simulink model "controlScheme_UDP_4Beads"  (R2019b)
settings: Solver=FixedStepAuto  StartTime=0.0  StopTime=Inf  FixedStep=1/300  RelTol=1e-3  EnableMultiTasking=on
InitFcn:
  | tb = twinbeam('147.32.86.177', 30000);
  | 
  | tb.tracker_init(4);
  | pause(2)
  | 
  | tb.coords_subs(30006);
  | pause(1)
StopFcn:
  | delete(tb);
  | 
  | gen_udp = udp('147.32.86.177', 30001);
  | fopen(gen_udp);
  | fwrite(gen_udp, uint8('d'));
  | fclose(gen_udp);
  | delete(gen_udp);
model workspace (MAT data in the model file):
  NumberOfBeads = Simulink.Parameter
  NumberOfBeads.Value = 1
  NumberOfBeads.DataType = 'auto'
  NumberOfBeads.Dimensions = [1 1]
undefined symbols (not defined in the file): DiscIntNeverNeededParam, Joystick, Standard_Devices, UDP_Protocol
libraries: sldrtlib x3
settings Model: SimulationMode=accelerator  EnablePacing=on  ParameterArgumentNames=NumberOfBeads  OrderedModelArguments=off  ExplicitPartitioning=on  Creator=marti  LastModifiedBy=marti
settings SolverCC: ConcurrentTasks=on  AutoInsertRateTranBlk=on  MinimalZcImpactIntegration=on
settings DebuggingCC: ReadBeforeWriteMsg=DisableAll  WriteAfterWriteMsg=DisableAll  WriteAfterReadMsg=DisableAll
settings ModelReferenceCC: UpdateModelReferenceTargets=IfOutOfDate
settings SFSimCC: SFSimEcho=off
settings RTWCC: Description=Simulink Desktop Real-Time  SystemTargetFile=sldrt.tlc  TemplateMakefile=sldrt.tmf  RTWCompilerOptimization=on
settings CodeAppCC: MaxIdLength=95
settings SimulinkDesktopRealTimeCC: TargetPreCompLibLocation=C:\Program Files\MATLAB\R2019b\toolbox\sldrt\lib\win64  PreserveStateflowLocalDataDimensions=off

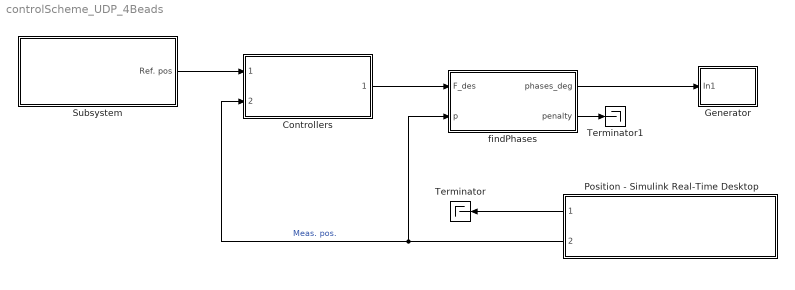
== system controlScheme_UDP_4Beads ==
  Controllers : Subsystem  TreatAsAtomicUnit=on  SystemSampleTime=1/30  ReferencedSubsystem=Controllers  P_const=300e-14  F_max=30e-11
  Generator : Subsystem  TreatAsAtomicUnit=on  SystemSampleTime=1/30
  Position - Simulink Real-Time Desktop : Subsystem  TreatAsAtomicUnit=on  SystemSampleTime=1/300  VariantControl=(default)  ReferencedSubsystem=UDP_position_subsystem  N_objs=4
  Subsystem : Subsystem  TreatAsAtomicUnit=on
  Terminator : Terminator
  Terminator1 : Terminator
  findPhases : MATLAB Function  TreatAsAtomicUnit=on  SystemSampleTime=1/30
  wires:
  Controllers/1 -> findPhases/1(F_des)
  Position - Simulink Real-Time Desktop/2 -> findPhases/2(p), Controllers/2  "Meas. pos."
  findPhases/1(phases_deg) -> Generator/1(In1)
  Position - Simulink Real-Time Desktop/1 -> Terminator/1
  Subsystem/1(Ref. pos) -> Controllers/1
  findPhases/2(penalty) -> Terminator1/1

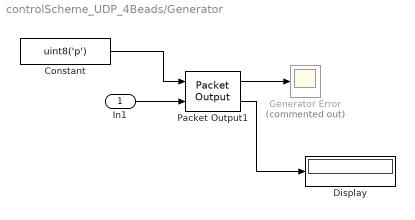
== system controlScheme_UDP_4Beads/Generator ==
  In1 : Inport
  Constant : Constant  Value=uint8('p')
  Display : Display
  Generator Error : Scope  Commented=on
  Packet Output1 : sldrtlib/Packet Output  SampleTime=1/30  MaxMissedTicks=400  ShowMissedTicks=on  YieldWhenWaiting=off  DrvName=Standard_Devices/UDP_Protocol  DrvAddress=30001  DrvOptions=[0 30001 49 52 55 46 51 50 46 56 54 46 49 55 55 0 0 0 0 0 0 0 0 0 0 0 0 0 0 0 0 0 0 0 0 0 0 0 0 0 0 0 0 0 0 0 0 0 0 0 0 0 0 0 0 0 0 0 0 0 0 0 0 0 0 0 0 0 0 0 0 0 0 0 0 0 0 0 0 0 0 0 0 0 0 0 0 0 0 0 0 0 0 0 0 0 0 0 0 0 0 0 0 0 0 0 0 0 0 0 0 0 0 0 0 0 0 0 0 0 0 0 0 0 0 0 0 0 0 0 0 0 0 0 0 0 0 0 0 0 0 0 0 0 0 0 0 0 0 0 0 0 0 0 0 0 0 0 0 0 0 0 0 0 0 0 0 0 0 0 0 0 0 0 0 0 0 0 0 0 0 0 0 0 0 0 0 0 0 0 0 0 0 0 0 0 0 0 0 0 0 0 0 0 0 0 0 0 0 0 0 0 0 0 0 0 0 0 0 0 0 0 0 0 0 0 0 0 0 0 0 0 0 0 0 0 0 0 0 0 0 0 0 0 0 0 0 0 0 0 0 0 0 0 0 0]  PacketSize=56*2+1  DataTypes={'uint8', '56*uint16'}  ShowReady=off  ShowError=on  PacketID=1  ByteOrder=1  InitialValue=[]  FinalValue=[]
      settings: AttributesFormatString=UDP Protocol [30001]
  wires:
  In1/1 -> Packet Output1/2
  Packet Output1/1 -> Generator Error/1
  Constant/1 -> Packet Output1/1
  Packet Output1/2 -> Display/1

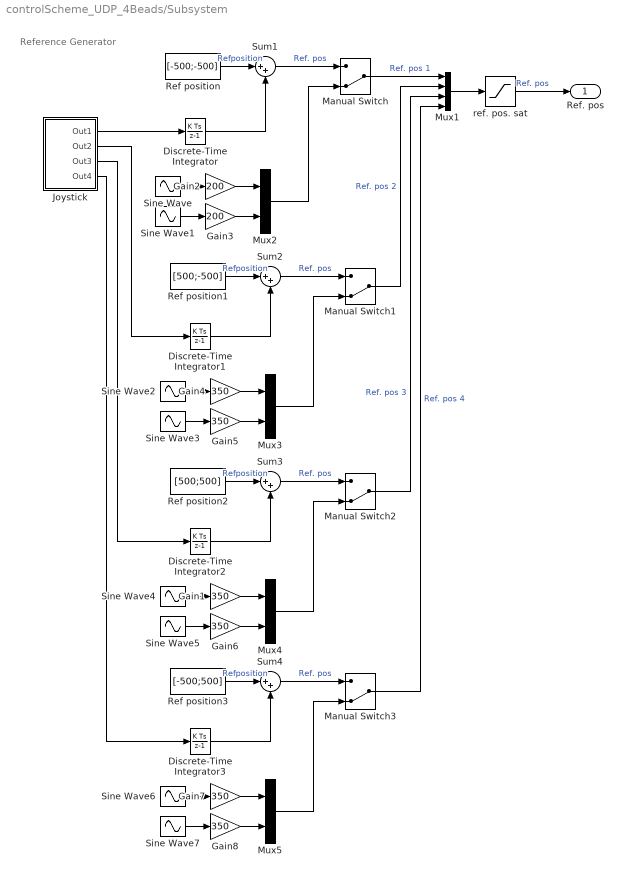
== system controlScheme_UDP_4Beads/Subsystem ==
  note: Reference Generator
  Discrete-Time Integrator{,1..3} (4 alike) : DiscreteIntegrator  gainval=1  SampleTime=-1  ICPrevOutput=DiscIntNeverNeededParam  ICPrevScaledInput=DiscIntNeverNeededParam
  Gain{1,4..8} (6 alike) : Gain  Gain=350
  Gain2 : Gain  Gain=200
  Gain3 : Gain  Gain=200
  Joystick : Subsystem
  Manual Switch{,1..3} (4 alike) : ManualSwitch  CurrentSetting=0
  Mux1 : Mux
  Mux{2..5} (4 alike) : Mux  Inputs=2
  Ref position : Constant  Value=[-500;-500]
  Ref position1 : Constant  Value=[500;-500]
  Ref position2 : Constant  Value=[500;500]
  Ref position3 : Constant  Value=[-500;500]
  Sine Wave : Sin  Frequency=2*pi/40  SampleTime=1/30
  Sine Wave1 : Sin  Frequency=2*pi/40  Phase=pi/2  SampleTime=1/30
  Sine Wave2 : Sin  Frequency=2*pi/40  Phase=2*pi/4  SampleTime=1/30
  Sine Wave3 : Sin  Frequency=2*pi/40  Phase=pi/2 + 2*pi/4  SampleTime=1/30
  Sine Wave4 : Sin  Frequency=2*pi/40  Phase=2*2*pi/4  SampleTime=1/30
  Sine Wave5 : Sin  Frequency=2*pi/40  Phase=pi/2 + 2*pi/4  SampleTime=1/30
  Sine Wave6 : Sin  Frequency=2*pi/40  Phase=3*pi/4  SampleTime=1/30
  Sine Wave7 : Sin  Frequency=2*pi/40  Phase=pi/2 + 3*pi/4  SampleTime=1/30
  Sum{1..4} (4 alike) : Sum  Inputs=|++
  ref. pos. sat : Saturate  UpperLimit=600  LowerLimit=-600
  Ref. pos : Outport
  wires:
  Sum2/1 -> Manual Switch1/1  "Ref. pos"
  Gain3/1 -> Mux2/2
  Gain6/1 -> Mux4/2
  Manual Switch1/1 -> Mux1/2  "Ref. pos 2"
  Joystick/4(Out4) -> Discrete-Time Integrator3/1
  Mux4/1 -> Manual Switch2/2
  Sine Wave3/1 -> Gain5/1
  Ref position/1 -> Sum1/1  "Refposition"
  Sine Wave5/1 -> Gain6/1
  Ref position1/1 -> Sum2/1  "Refposition"
  Manual Switch2/1 -> Mux1/3  "Ref. pos 3"
  Joystick/1(Out1) -> Discrete-Time Integrator/1
  Ref position2/1 -> Sum3/1  "Refposition"
  Discrete-Time Integrator2/1 -> Sum3/2
  Sine Wave4/1 -> Gain1/1
  Gain8/1 -> Mux5/2
  Sum3/1 -> Manual Switch2/1  "Ref. pos"
  Joystick/3(Out3) -> Discrete-Time Integrator2/1
  Manual Switch3/1 -> Mux1/4  "Ref. pos 4"
  Gain4/1 -> Mux3/1
  Gain5/1 -> Mux3/2
  Sine Wave1/1 -> Gain3/1
  Mux2/1 -> Manual Switch/2
  Sum4/1 -> Manual Switch3/1  "Ref. pos"
  Gain1/1 -> Mux4/1
  Discrete-Time Integrator/1 -> Sum1/2
  Discrete-Time Integrator1/1 -> Sum2/2
  Mux3/1 -> Manual Switch1/2
  Sine Wave/1 -> Gain2/1
  ref. pos. sat/1 -> Ref. pos/1  "Ref. pos"
  Sine Wave2/1 -> Gain4/1
  Mux1/1 -> ref. pos. sat/1
  Gain2/1 -> Mux2/1
  Manual Switch/1 -> Mux1/1  "Ref. pos 1"
  Ref position3/1 -> Sum4/1  "Refposition"
  Sum1/1 -> Manual Switch/1  "Ref. pos"
  Joystick/2(Out2) -> Discrete-Time Integrator1/1
  Discrete-Time Integrator3/1 -> Sum4/2
  Sine Wave7/1 -> Gain8/1
  Mux5/1 -> Manual Switch3/2
  Gain7/1 -> Mux5/1
  Sine Wave6/1 -> Gain7/1

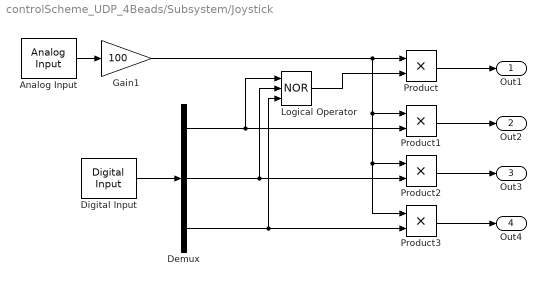
== system controlScheme_UDP_4Beads/Subsystem/Joystick ==
  Analog Input : sldrtlib/Analog Input  SampleTime=1/30  MaxMissedTicks=200  ShowMissedTicks=off  YieldWhenWaiting=off  DrvName=Standard_Devices/Joystick  DrvAddress=1  DrvOptions=zeros(1,0)  Channels=[1:2]  RangeMode=1  VoltRange=1  DataType=1
      settings: AttributesFormatString=Joystick [1]
  Demux : Demux  Outputs=3
  Digital Input : sldrtlib/Digital Input  SampleTime=1/30  MaxMissedTicks=200  ShowMissedTicks=off  YieldWhenWaiting=off  DrvName=Standard_Devices/Joystick  DrvAddress=1  DrvOptions=zeros(1,0)  Channels=1:3  BitMode=1  DataType=9
      settings: AttributesFormatString=Joystick [1]  SourceProductBaseCode=WT
  Gain1 : Gain  Gain=100
  Logical Operator : Logic  Operator=NOR  Inputs=3  AllPortsSameDT=off  OutDataTypeStr=boolean
  Product{,1..3} (4 alike) : Product
  Out1 : Outport
  Out2 : Outport  Port=2
  Out3 : Outport  Port=3
  Out4 : Outport  Port=4
  wires:
  Product1/1 -> Out2/1
  Logical Operator/1 -> Product/2
  Product/1 -> Out1/1
  Demux/1 -> Logical Operator/1, Product1/2
  Analog Input/1 -> Gain1/1
  Gain1/1 -> Product/1, Product3/1, Product2/1, Product1/1
  Digital Input/1 -> Demux/1
  Demux/2 -> Logical Operator/2, Product2/2
  Product2/1 -> Out3/1
  Product3/1 -> Out4/1
  Demux/3 -> Logical Operator/3, Product3/2

== matlab function controlScheme_UDP_4Beads/findPhases ==
  data: F_des input; p input; phases_deg output; penalty output
function [phases_deg, penalty] = fcn(F_des, p)
[phases_rad, penalty] = findPhasesFoGivenF(p*1e-6, F_des);
phases_deg = rad2deg(phases_rad);
phases_deg = round(mod(phases_deg, 360));
